simulink library "openLoopCtrl_cl"  (R2018a)
settings: Solver=VariableStepAuto  StartTime=0.0  StopTime=10.0  RelTol=1e-3
libraries: pathProjection_ul x1
settings Model: Creator=mcobb  LastModifiedBy=mcobb

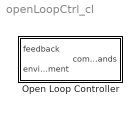
== system openLoopCtrl_cl ==
  Open Loop Controller : Subsystem  VariantControl=VSS_OPENLOOP_CTRL

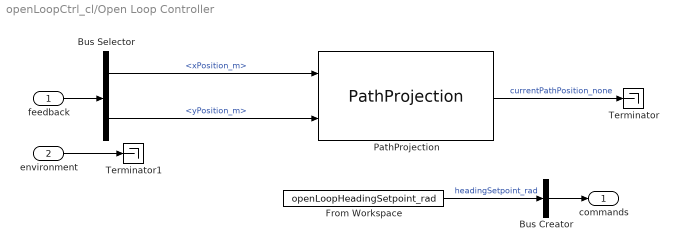
== system openLoopCtrl_cl/Open Loop Controller ==
  feedback : Inport
  environment : Inport  Port=2
  Bus Creator : BusCreator  Inputs=1
  Bus Selector : BusSelector  OutputSignals=xPosition_m,yPosition_m
  From Workspace : FromWorkspace  VariableName=openLoopHeadingSetpoint_rad  SampleTime=0
  PathProjection : pathProjection_ul/PathProjection
  Terminator : Terminator
  Terminator1 : Terminator
  commands : Outport
  wires:
  environment/1 -> Terminator1/1
  From Workspace/1 -> Bus Creator/1  "headingSetpoint_rad"
  Bus Creator/1 -> commands/1
  feedback/1 -> Bus Selector/1
  Bus Selector/1 -> PathProjection/1  "<xPosition_m>"
  Bus Selector/2 -> PathProjection/2  "<yPosition_m>"
  PathProjection/1 -> Terminator/1  "currentPathPosition_none"
